simulink model "USV_SASTnewlaw_env"  (R2023a)
settings: Solver=ode4  StartTime=0.0  StopTime=60  FixedStep=0.01  RelTol=1e-3
undefined symbols (not defined in the file or in its folder): sigbuilder_block
libraries: sharedutil x6, simulink_extras x1, aerolibutil x1
(part 1 of 2)
settings Model: Creator=Alex Glz  LastModifiedBy=maxpr
settings SolverCC: ZeroCrossAlgorithm=Adaptive  AlgebraicLoopSolver=TrustRegion
settings DataIOCC: ReturnWorkspaceOutputs=off
settings DebuggingCC: IgnoredZcDiagnostic=none  UnconnectedInputMsg=warning  UnconnectedOutputMsg=warning  UnconnectedLineMsg=warning  PregeneratedLibrarySubsystemCodeDiagnostic=none  ArithmeticOperatorsInVariantConditions=warning
settings ModelReferenceCC: EnableRefExpFcnMdlSchedulingChecks=on
settings SFSimCC: SimUseLocalCustomCode=off  CustomCodeUndefinedFunction=UseInterfaceOnly
settings RTWCC: RTWUseLocalCustomCode=off

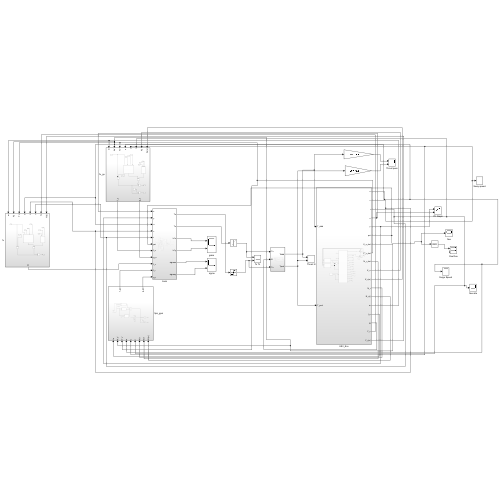
[thumbnail: Simulink's stored preview of the top-level diagram]
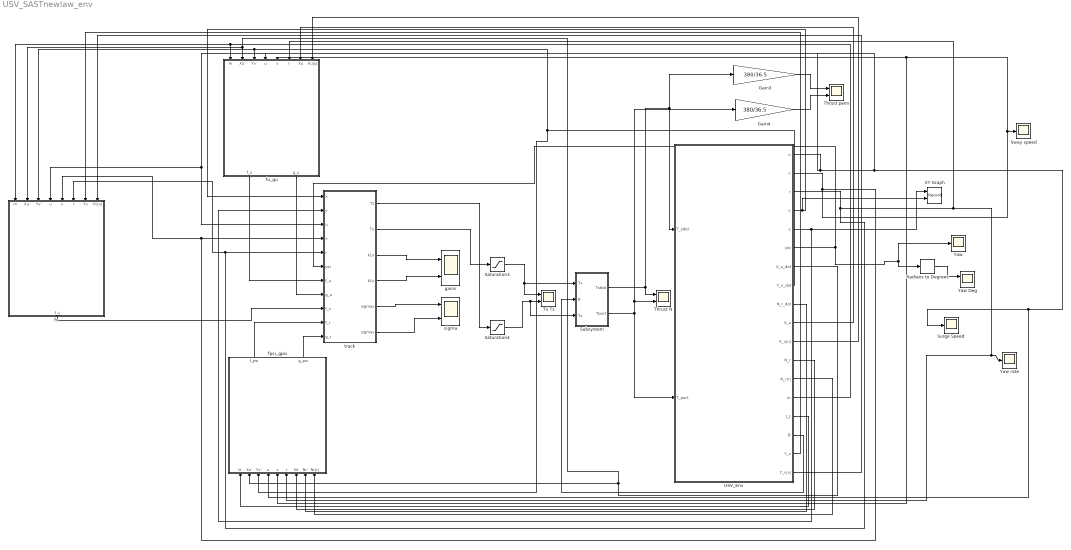
== system USV_SASTnewlaw_env ==
  Gain3 : Gain  Gain=380/36.5
  Gain4 : Gain  Gain=380/36.5
  Radians to Degrees : simulink_extras/Transformations/Radians to Degrees
  Saturation3 : Saturate  UpperLimit=64.97  LowerLimit=-64.97
  Saturation4 : Saturate  UpperLimit=13.31  LowerLimit=-13.31
  Subsystem : Subsystem
  Surge Speed : Scope
  Sway speed : Scope
  Thrust N : Scope  NumInputPorts=2
  Thrust pwm : Scope  NumInputPorts=2
  Tx Tz : Scope  NumInputPorts=2
  USV_Env : Subsystem
  XY Graph : Record  FileSettingsInternal="{\"entries\":[{\"content\":{\"excelSettings\":{\"content\":{},\"type\":\"Streamout.ExcelSettings\"}},\"type\":\"Streamout.FileSettingStorage\",\"uuid\":\"\"}],\"packageUris\":[\"http:\\/\\/schema.mathworks.com\\/mf0\\/streamout_blocks\\/R2020a\"],\"version\":\"1.0\"}"  Layout=[1 1]  SignalsInternal="{\"entries\":[{\"content\":{\"signals\":[{\"content\":{\"blockPath\":[],\"dimensions\":[1],\"domain\":\"\",\"lineColor\":\"#a2142f\",\"plots\":[1],\"port\":1,\"sid\":[\"\"],\"signalID\":306,\"signalName\":\"USV_Env:5\"},\"type\":\"RecordBlkView.Signal\",\"uuid\":\"\"},{\"content\":{\"blockPath\":[],\"dimensions\":[1],\"domain\":\"\",\"lineColor\":\"#139fff\",\"plots\":[1],\"port\":2,\"sid\":[\"\"],\"signalID\":310,\"signalName\":\"USV_Env:4\"},\"type\":\"RecordBlkView.Signal\",\"uuid\":\"\"}]},\"type\":\"RecordBlkView.InputSignals\",\"uuid\":\"\"}],\"packageUris\":[\"http:\\/\\/schema.mathworks.com\\/mf0\\/streamout_blocks\\/R2020a\"],\"version\":\"1.0\"}"  VisualizationBindings="{\"xyplotplugin\":{\"info\":[{\"series\":[{\"bindingParametersList\":[{\"parameter\":\"X-Axis\",\"signalID\":306,\"signalName\":\"USV_Env:5\"},{\"parameter\":\"Y-Axis\",\"signalID\":310,\"signalName\":\"USV_Env:4\"}],\"seriesID\":45570}],\"subplotID\":1}]}}"  CompatibilityTag=XY  st=-1
  Yaw : Scope
  Yaw Deg : Scope  NumInputPorts=2
  Yaw rate : Scope
  fpsi_gpsi : Subsystem
  fu_gu : Subsystem
  fv : Subsystem
  gains : Scope  NumInputPorts=2
  sigma : Scope  NumInputPorts=2
  track : Subsystem
  wires:
  Gain4/1 -> Thrust pwm/2
  Gain3/1 -> Thrust pwm/1
  USV_Env/16(B) -> Subsystem/2(B)
  USV_Env/14(m) -> fv/1(m), fu_gu/1(m)
  USV_Env/7(X_u_dot) -> fv/2(Xu'), fu_gu/2(Xu'), fpsi_gpsi/2(Xu')
  USV_Env/8(Y_v_dot) -> fpsi_gpsi/3(Yv'), fv/3(Yv'), fu_gu/3(Yv')
  USV_Env/1(u) -> fpsi_gpsi/4(u), Surge Speed/1, fu_gu/4(u), track/3(u), fv/4(u)
  USV_Env/2(v) -> fpsi_gpsi/5(v), fu_gu/5(v), Sway speed/1, fv/5(v), track/4(v)
  USV_Env/3(r) -> fv/6(r), track/5(r), fpsi_gpsi/6(r), Yaw rate/1, fu_gu/6(r)
  USV_Env/10(X_u) -> fu_gu/7(Xu)
  USV_Env/11(X_u|u|) -> fu_gu/8(Xu|u|)
  USV_Env/15(I_z) -> fpsi_gpsi/1(Iz)
  USV_Env/12(N_r) -> fpsi_gpsi/7(Nr)
  USV_Env/9(N_r_dot) -> fpsi_gpsi/8(Nr')
  USV_Env/5(y) -> track/2(y), XY Graph/1
  USV_Env/4(x) -> track/1(x), XY Graph/2
  Radians to Degrees/1 -> Yaw Deg/1
  USV_Env/6(psi) -> Yaw/1, Radians to Degrees/1, track/6(psi)
  Saturation4/1 -> Subsystem/3(Tz), Tx Tz/2
  Saturation3/1 -> Subsystem/1(Tx), Tx Tz/1
  Subsystem/2(Tport) -> USV_Env/2(T_port), Thrust N/2, Gain4/1
  Subsystem/1(Tstbd) -> Thrust N/1, USV_Env/1(T_stbd), Gain3/1
  USV_Env/13(N_r|r|) -> fpsi_gpsi/9(Nr|r|)
  track/3(k1x) -> gains/1
  track/4(k1y) -> gains/2
  track/5(sigmax) -> sigma/1
  track/6(sigmay) -> sigma/2
  track/2(Tx) -> Saturation3/1
  track/1(Tz) -> Saturation4/1
  fpsi_gpsi/1(f_psi) -> track/10(f_r)
  fpsi_gpsi/2(g_psi) -> track/11(g_r)
  fu_gu/1(f_u) -> track/7(f_u)
  fu_gu/2(g_u) -> track/8(g_u)
  USV_Env/17(Y_v) -> fv/7(Yv)
  USV_Env/18(Y_v|v|) -> fv/8(Yv|v|)
  fv/1(f_v) -> track/9(f_v)

== system USV_SASTnewlaw_env/Subsystem ==
  Tx : Inport
  B : Inport  Port=2
  Tz : Inport  Port=3
  Gain : Gain  Gain=1/2
  Gain1 : Gain  Gain=1/2
  Product : Product  Inputs=*/
  Product1 : Product  Inputs=*/
  Saturation1 : Saturate  UpperLimit=36.5  LowerLimit=-30
  Saturation2 : Saturate  UpperLimit=36.5  LowerLimit=-30
  Sum : Sum
  Sum1 : Sum  Inputs=+-
  Tstbd : Outport  VectorParamsAs1DForOutWhenUnconnected=off
  Tport : Outport  Port=2  VectorParamsAs1DForOutWhenUnconnected=off
  wires:
  Sum1/1 -> Saturation2/1
  Gain/1 -> Sum/1
  Sum/1 -> Saturation1/1
  B/1 -> Product/2, Product1/2
  Tz/1 -> Product1/1, Product/1
  Saturation1/1 -> Tport/1
  Product/1 -> Sum/2
  Tx/1 -> Gain1/1, Gain/1
  Product1/1 -> Sum1/2
  Saturation2/1 -> Tstbd/1
  Gain1/1 -> Sum1/1

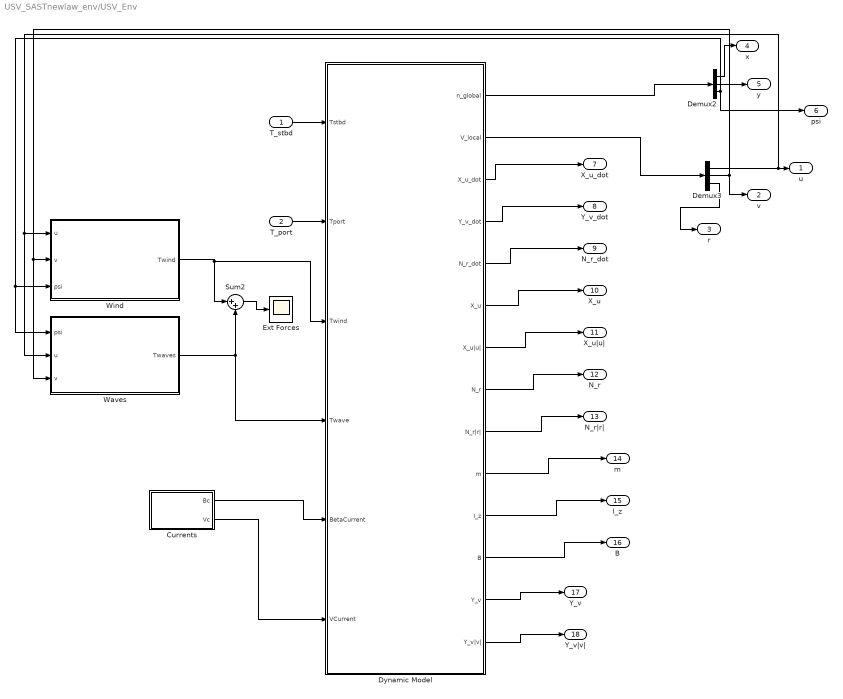
== system USV_SASTnewlaw_env/USV_Env ==
  T_stbd : Inport
  T_port : Inport  Port=2
  Currents : Subsystem
  Demux2 : Demux  Outputs=3
  Demux3 : Demux  Outputs=3
  Dynamic Model : Subsystem
  Ext Forces : Scope
  Sum2 : Sum  Inputs=|++
  Waves : Subsystem
  Wind : Subsystem
  u : Outport
  v : Outport  Port=2
  r : Outport  Port=3
  x : Outport  Port=4
  y : Outport  Port=5
  psi : Outport  Port=6
  X_u_dot : Outport  Port=7  VectorParamsAs1DForOutWhenUnconnected=off
  Y_v_dot : Outport  Port=8  VectorParamsAs1DForOutWhenUnconnected=off
  N_r_dot : Outport  Port=9  VectorParamsAs1DForOutWhenUnconnected=off
  X_u : Outport  Port=10  VectorParamsAs1DForOutWhenUnconnected=off
  X_u|u| : Outport  Port=11  VectorParamsAs1DForOutWhenUnconnected=off
  N_r : Outport  Port=12  VectorParamsAs1DForOutWhenUnconnected=off
  N_r|r| : Outport  Port=13  VectorParamsAs1DForOutWhenUnconnected=off
  m : Outport  Port=14  VectorParamsAs1DForOutWhenUnconnected=off
  I_z : Outport  Port=15  VectorParamsAs1DForOutWhenUnconnected=off
  B : Outport  Port=16  VectorParamsAs1DForOutWhenUnconnected=off
  Y_v : Outport  Port=17  VectorParamsAs1DForOutWhenUnconnected=off
  Y_v|v| : Outport  Port=18  VectorParamsAs1DForOutWhenUnconnected=off
  wires:
  T_stbd/1 -> Dynamic Model/1(Tstbd)
  Currents/1(Bc) -> Dynamic Model/5(BetaCurrent)
  T_port/1 -> Dynamic Model/2(Tport)
  Dynamic Model/2(V_local) -> Demux3/1
  Demux3/2 -> v/1, Waves/3(v), Wind/2(v)
  Demux2/3 -> psi/1, Waves/1(psi), Wind/3(psi)
  Dynamic Model/1(n_global) -> Demux2/1
  Demux3/1 -> u/1, Waves/2(u), Wind/1(u)
  Currents/2(Vc) -> Dynamic Model/6(VCurrent)
  Demux3/3 -> r/1
  Demux2/1 -> x/1
  Demux2/2 -> y/1
  Dynamic Model/3(X_u_dot) -> X_u_dot/1
  Dynamic Model/4(Y_v_dot) -> Y_v_dot/1
  Dynamic Model/5(N_r_dot) -> N_r_dot/1
  Dynamic Model/6(X_u) -> X_u/1
  Dynamic Model/7(X_u|u|) -> X_u|u|/1
  Dynamic Model/8(N_r) -> N_r/1
  Dynamic Model/9(N_r|r|) -> N_r|r|/1
  Dynamic Model/11(I_z) -> I_z/1
  Dynamic Model/10(m) -> m/1
  Dynamic Model/12(B) -> B/1
  Waves/1(Twaves) -> Dynamic Model/4(Twave), Sum2/2
  Wind/1(Twind) -> Dynamic Model/3(Twind), Sum2/1
  Sum2/1 -> Ext Forces/1
  Dynamic Model/13(Y_v) -> Y_v/1
  Dynamic Model/14(Y_v|v|) -> Y_v|v|/1

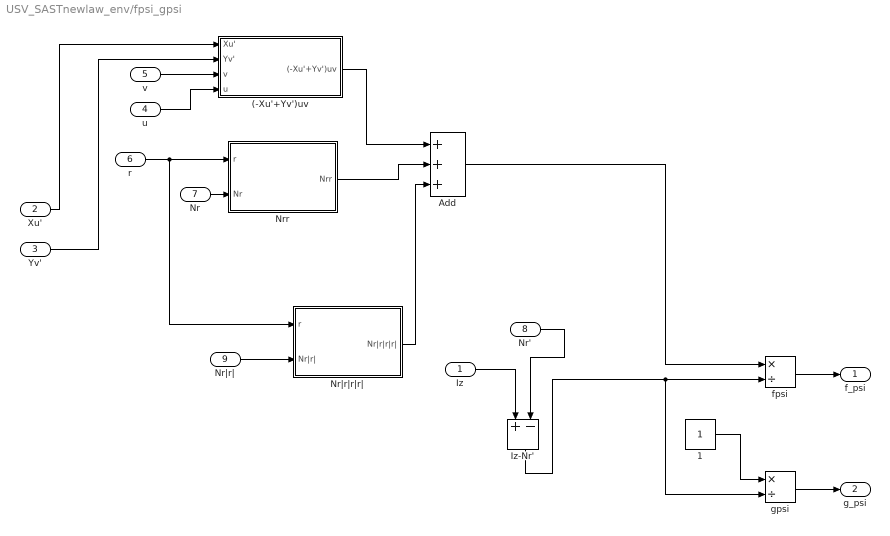
== system USV_SASTnewlaw_env/fpsi_gpsi ==
  Iz : Inport
  Xu' : Inport  Port=2
  Yv' : Inport  Port=3
  u : Inport  Port=4
  v : Inport  Port=5
  r : Inport  Port=6
  Nr : Inport  Port=7
  Nr' : Inport  Port=8
  Nr|r| : Inport  Port=9
  (-Xu'+Yv')uv : Subsystem
  1 : Constant  SampleTime=Inf
  Add : Sum  Inputs=+++
  Iz-Nr' : Sum  Inputs=+-
  Nrr : Subsystem
  Nr|r|r|r| : Subsystem
  fpsi : Product  Inputs=*/
  gpsi : Product  Inputs=*/
  f_psi : Outport  VectorParamsAs1DForOutWhenUnconnected=off
  g_psi : Outport  Port=2  VectorParamsAs1DForOutWhenUnconnected=off
  wires:
  Nr/1 -> Nrr/2(Nr)
  Yv'/1 -> (-Xu'+Yv')uv/2(Yv')
  r/1 -> Nrr/1(r), Nr|r|r|r|/1(r)
  (-Xu'+Yv')uv/1((-Xu'+Yv')uv) -> Add/1
  v/1 -> (-Xu'+Yv')uv/3(v)
  Iz/1 -> Iz-Nr'/1
  Nrr/1(Nrr) -> Add/2
  u/1 -> (-Xu'+Yv')uv/4(u)
  Xu'/1 -> (-Xu'+Yv')uv/1(Xu')
  Nr'/1 -> Iz-Nr'/2
  Nr|r|/1 -> Nr|r|r|r|/2(Nr|r|)
  Nr|r|r|r|/1(Nr|r|r|r|) -> Add/3
  1/1 -> gpsi/1
  gpsi/1 -> g_psi/1
  fpsi/1 -> f_psi/1
  Iz-Nr'/1 -> gpsi/2, fpsi/2
  Add/1 -> fpsi/1

== system USV_SASTnewlaw_env/fu_gu ==
  m : Inport
  Xu' : Inport  Port=2
  Yv' : Inport  Port=3
  u : Inport  Port=4
  v : Inport  Port=5
  r : Inport  Port=6
  Xu : Inport  Port=7
  Xu|u| : Inport  Port=8
  (m-Yv')vr : Subsystem
  1 : Constant  SampleTime=Inf
  Xdrag : Subsystem
  fu : Product  Inputs=*/
  fu*gu : Sum
  gu : Product  Inputs=*/
  m-Xu' : Sum  Inputs=+-
  f_u : Outport  VectorParamsAs1DForOutWhenUnconnected=off
  g_u : Outport  Port=2  VectorParamsAs1DForOutWhenUnconnected=off
  wires:
  Xu/1 -> Xdrag/2(Xu)
  Yv'/1 -> (m-Yv')vr/2(Yv')
  r/1 -> (m-Yv')vr/4(r)
  Xu|u|/1 -> Xdrag/3(Xu|u|)
  m-Xu'/1 -> gu/2, fu/2
  v/1 -> (m-Yv')vr/3(v)
  m/1 -> (m-Yv')vr/1(m), m-Xu'/1
  u/1 -> Xdrag/1(u)
  Xu'/1 -> m-Xu'/2
  (m-Yv')vr/1((m-Yv')vr) -> fu*gu/1
  Xdrag/1(Xdrag) -> fu*gu/2
  fu*gu/1 -> fu/1
  fu/1 -> f_u/1
  gu/1 -> g_u/1
  1/1 -> gu/1

== system USV_SASTnewlaw_env/fv ==
  m : Inport
  Xu' : Inport  Port=2
  Yv' : Inport  Port=3
  u : Inport  Port=4
  v : Inport  Port=5
  r : Inport  Port=6
  Yv : Inport  Port=7
  Yv|v| : Inport  Port=8
  (m-Yv')vr : Subsystem
  Xur + Yuv : Sum
  Ydrag : Subsystem
  fv : Product  Inputs=*/
  m-Yv' : Sum  Inputs=+-
  f_v : Outport  VectorParamsAs1DForOutWhenUnconnected=off
  wires:
  Yv/1 -> Ydrag/2(Yv)
  Yv'/1 -> m-Yv'/2
  r/1 -> (m-Yv')vr/4(r)
  Yv|v|/1 -> Ydrag/3(Yv|v|)
  m-Yv'/1 -> fv/2
  v/1 -> Ydrag/1(v)
  m/1 -> (m-Yv')vr/1(m), m-Yv'/1
  u/1 -> (m-Yv')vr/3(u)
  Xu'/1 -> (m-Yv')vr/2(Xu')
  fv/1 -> f_v/1
  Xur + Yuv/1 -> fv/1
  (m-Yv')vr/1((-m+Xu')ur) -> Xur + Yuv/1
  Ydrag/1(Ydrag) -> Xur + Yuv/2

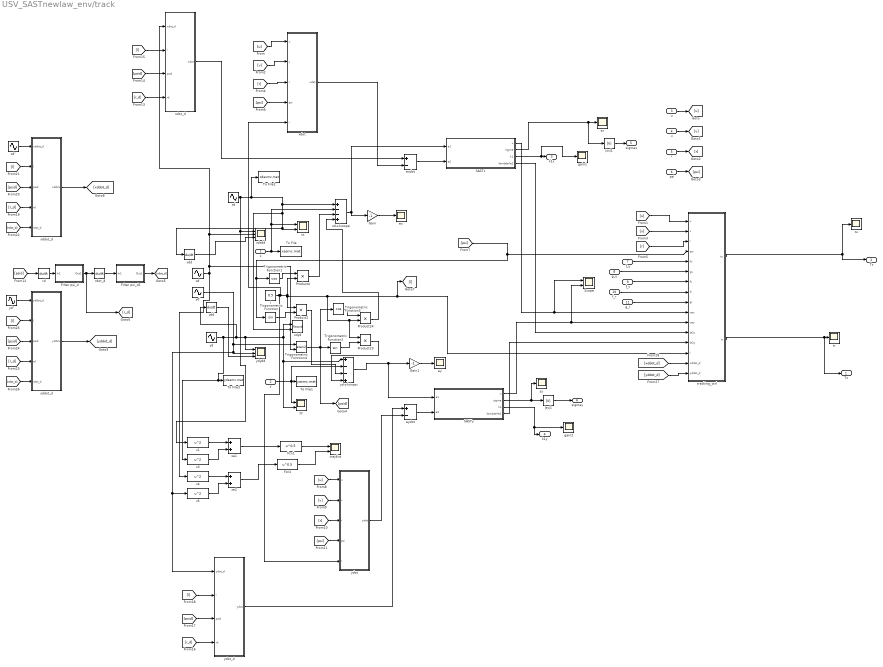
== system USV_SASTnewlaw_env/track ==
  x : Inport
  y : Inport  Port=2
  u : Inport  Port=3
  v : Inport  Port=4
  r : Inport  Port=5
  psi : Inport  Port=6
  f_u : Inport  Port=7
  g_u : Inport  Port=8
  f_v : Inport  Port=9
  f_r : Inport  Port=10
  g_r : Inport  Port=11
  Fcn1 : Fcn  Expr=u^0.5
  Fcn2 : Fcn  Expr=u^0.5
  Filter psi_d : Subsystem
  Filter psi_d1 : Subsystem
  Gain : Gain  Gain=-1
  Gain1 : Gain  Gain=-1
  Product{2,4,23..24} (4 alike) : Product
  SASTx : Subsystem
  SASTy : Subsystem
  Scope : Scope  NumInputPorts=2
  To File : ToFile  Filename=xasmc.mat
  To File1 : ToFile  Filename=yasmc.mat
  To File2 : ToFile  Filename=xdasmc.mat
  To File3 : ToFile  Filename=ydasmc.mat
  Trigonometric Function : Trigonometry
  Trigonometric Function1 : Trigonometry  Operator=cos
  Trigonometric Function2 : Trigonometry
  Trigonometric Function3 : Trigonometry  Operator=cos
  Trigonometric Function4 : Trigonometry  Operator=atan2
  ex : Scope
  exdot : Sum  Inputs=+-
  ey : Scope
  eydot : Sum  Inputs=+-
  gain1 : Scope
  gain2 : Scope
  l : Constant  Value=0.5
  rd : Derivative
  rdot_d : Derivative
  sx : Scope
  sy : Scope
  tr : Scope
  tracking_ctrl : MATLAB Function  TreatAsAtomicUnit=on
  trajdist : Scope  NumInputPorts=2
  tu : Scope
  v{1,3..5} (4 alike) : Fcn  Expr=u^2
  xd : Sin  Amplitude=2.5  Bias=0.5  Frequency=pi/15  SampleTime=0
  xd' : Sin  Amplitude=2.5*pi/15  Frequency=pi/15  Phase=pi/2  SampleTime=0
  xd'' : Sin  Amplitude=-2.5*(pi/15)*(pi/15)  Frequency=pi/15  SampleTime=0
  xd-x-lcospsi : Sum  Inputs=+--+
  xdd : Derivative
  xddot_d : MATLAB Function  TreatAsAtomicUnit=on
  xdot : MATLAB Function  TreatAsAtomicUnit=on
  xdot_d : MATLAB Function  TreatAsAtomicUnit=on
  xdxdd : Scope  NumInputPorts=3
  xdyd : Record  FileSettingsInternal="{\"entries\":[{\"content\":{\"excelSettings\":{\"content\":{},\"type\":\"Streamout.ExcelSettings\"}},\"type\":\"Streamout.FileSettingStorage\",\"uuid\":\"\"}],\"packageUris\":[\"http:\\/\\/schema.mathworks.com\\/mf0\\/streamout_blocks\\/R2020a\"],\"version\":\"1.0\"}"  Layout=[1 1]  SignalsInternal="{\"entries\":[{\"content\":{\"signals\":[{\"content\":{\"blockPath\":[],\"dimensions\":[1],\"domain\":\"\",\"lineColor\":\"#a2142f\",\"plots\":[1],\"port\":1,\"sid\":[\"\"],\"signalID\":395,\"signalName\":\"yd\"},\"type\":\"RecordBlkView.Signal\",\"uuid\":\"\"},{\"content\":{\"blockPath\":[],\"dimensions\":[1],\"domain\":\"\",\"lineColor\":\"#139fff\",\"plots\":[1],\"port\":2,\"sid\":[\"\"],\"signalID\":399,\"signalName\":\"xd\"},\"type\":\"RecordBlkView.Signal\",\"uuid\":\"\"}]},\"type\":\"RecordBlkView.InputSignals\",\"uuid\":\"\"}],\"packageUris\":[\"http:\\/\\/schema.mathworks.com\\/mf0\\/streamout_blocks\\/R2020a\"],\"version\":\"1.0\"}"  VisualizationBindings="{\"xyplotplugin\":{\"info\":[{\"series\":[{\"bindingParametersList\":[{\"parameter\":\"X-Axis\",\"signalID\":395,\"signalName\":\"yd\"},{\"parameter\":\"Y-Axis\",\"signalID\":399,\"signalName\":\"xd\"}],\"seriesID\":16886}],\"subplotID\":1}]}}"  CompatibilityTag=XY  st=-1
  xe1 : Sum
  xe2 : Sum
  xx : Scope  NumInputPorts=2
  yd : Sin  Amplitude=7  Bias=-7.5  Frequency=pi/30  Phase=pi/2  SampleTime=0
  yd' : Sin  Amplitude=-7*pi/30  Frequency=pi/30  SampleTime=0
  yd'' : Sin  Amplitude=-7*(pi/30)*(pi/30)  Frequency=pi/30  Phase=pi/2  SampleTime=0
  yd-y-lsinpsi : Sum  Inputs=+--+
  ydd : Derivative
  yddot_d : MATLAB Function  TreatAsAtomicUnit=on
  ydot : MATLAB Function  TreatAsAtomicUnit=on
  ydot_d : MATLAB Function  TreatAsAtomicUnit=on
  ydydd : Scope  NumInputPorts=3
  yy : Scope  NumInputPorts=2
  |sx|1 : Abs  SaturateOnIntegerOverflow=off
  |sy|1 : Abs  SaturateOnIntegerOverflow=off
  Tz : Outport
  Tx : Outport  Port=2
  k1x : Outport  Port=3  VectorParamsAs1DForOutWhenUnconnected=off
  k1y : Outport  Port=4  VectorParamsAs1DForOutWhenUnconnected=off
  sigmax : Outport  Port=5  VectorParamsAs1DForOutWhenUnconnected=off
  sigmay : Outport  Port=6  VectorParamsAs1DForOutWhenUnconnected=off
  wires:
  tracking_ctrl/2(tr) -> Tz/1, tr/1
  y/1 -> yd-y-lsinpsi/2, To File1/1, yy/1
  x/1 -> xd-x-lcospsi/2, xx/1, To File/1
  xd/1 -> v1/1, xdxdd/1, To File2/1, xd-x-lcospsi/1, xx/2, xdd/1, xdyd/2
  yd/1 -> v3/1, To File3/1, yd-y-lsinpsi/1, yy/2, xdyd/1, ydydd/1, ydd/1
  xd-x-lcospsi/1 -> SASTx/1(e1), Gain/1
  yd'/1 -> ydydd/2, ydot_d/1(ydot_d), v5/1, Trigonometric Function4/1
  xd'/1 -> xdot_d/1(xdot_d), xdxdd/2, Trigonometric Function4/2, v4/1
  tracking_ctrl/1(tu) -> tu/1, Tx/1
  ydd/1 -> ydydd/3
  xdd/1 -> xdxdd/3
  Fcn1/1 -> trajdist/1
  Fcn2/1 -> trajdist/2
  xe1/1 -> Fcn1/1
  v1/1 -> xe1/1
  v3/1 -> xe1/2
  xe2/1 -> Fcn2/1
  v4/1 -> xe2/1
  v5/1 -> xe2/2
  yd-y-lsinpsi/1 -> SASTy/1(e1), Gain1/1
  Product2/1 -> yd-y-lsinpsi/3
  Product4/1 -> xd-x-lcospsi/3
  [psi] -> tracking_ctrl/4(psi), Trigonometric Function1/1, Trigonometric Function/1
  Trigonometric Function1/1 -> Product4/1
  Trigonometric Function/1 -> Product2/2
  SASTx/2(sigma) -> |sx|1/1, sx/1
  |sy|1/1 -> sigmay/1
  |sx|1/1 -> sigmax/1
  Trigonometric Function4/1 -> Trigonometric Function3/1, Trigonometric Function2/1, [psid]
  Trigonometric Function2/1 -> Product23/2
  Trigonometric Function3/1 -> Product24/1
  Product23/1 -> yd-y-lsinpsi/4
  Product24/1 -> xd-x-lcospsi/4
  SASTx/3(k1) -> gain1/1, k1x/1
  SASTy/2(sigma) -> sy/1, |sy|1/1
  SASTy/3(k1) -> k1y/1, gain2/1
  u/1 -> [u]
  [v] -> tracking_ctrl/2(v)
  [r] -> tracking_ctrl/3(r)
  f_u/1 -> tracking_ctrl/5(fu)
  g_u/1 -> tracking_ctrl/6(gu)
  f_v/1 -> tracking_ctrl/7(fv)
  f_r/1 -> tracking_ctrl/8(fr)
  g_r/1 -> tracking_ctrl/9(gr)
  SASTx/1(u) -> tracking_ctrl/10(uax), Scope/1
  SASTy/1(u) -> tracking_ctrl/11(uay), Scope/2
  SASTx/4(lambda*e2) -> tracking_ctrl/12(le2x)
  SASTy/4(lambda*e2) -> tracking_ctrl/13(le2y)
  eydot/1 -> SASTy/2(e2)
  exdot/1 -> SASTx/2(e2)
  xdot/1(xdot) -> exdot/2
  [u] -> xdot/1(u)
  [u] -> tracking_ctrl/1(u)
  psi/1 -> [psi]
  v/1 -> [v]
  r/1 -> [r]
  [v] -> xdot/2(v)
  [r] -> xdot/3(r)
  [psi] -> xdot/4(psi)
  ydot/1(ydot) -> eydot/2
  [r] -> ydot/3(r)
  l/1 -> ydot/5(l), xdot/5(l), [l], tracking_ctrl/14(l), Product23/1, Product24/2, Product2/1, Product4/2
  [v] -> ydot/2(v)
  [psi] -> ydot/4(psi)
  [u] -> ydot/1(u)
  xdot_d/1(xdot) -> exdot/1
  [psid] -> rd/1
  rd/1 -> Filter psi_d/1(In1)
  rdot_d/1 -> Filter psi_d1/1(In1)
  [r_d] -> xdot_d/4(rd)
  [psid] -> xdot_d/3(psid)
  [l] -> xdot_d/2(l)
  ydot_d/1(ydot) -> eydot/1
  [l] -> ydot_d/2(l)
  [r_d] -> ydot_d/4(rd)
  [psid] -> ydot_d/3(psid)
  xd''/1 -> xddot_d/1(xddot_d)
  [l] -> xddot_d/2(l)
  [psid] -> xddot_d/3(psid)
  [r_d] -> xddot_d/4(rd)
  [rdot_d] -> xddot_d/5(rdot_d)
  xddot_d/1(xddot) -> [xddot_d]
  yddot_d/1(yddot) -> [yddot_d]
  [psid] -> yddot_d/3(psid)
  [l] -> yddot_d/2(l)
  [r_d] -> yddot_d/4(rd)
  [rdot_d] -> yddot_d/5(rdot_d)
  yd''/1 -> yddot_d/1(yddot_d)
  [yddot_d] -> tracking_ctrl/16(yddot_d)
  [xddot_d] -> tracking_ctrl/15(xddot_d)
  Filter psi_d/1(Out1) -> rdot_d/1, [r_d]
  Filter psi_d1/1(Out1) -> [rdot_d]
  Gain/1 -> ex/1
  Gain1/1 -> ey/1

== system USV_SASTnewlaw_env/USV_Env/Currents ==
  Beta : Constant  Value=0.8
  Current Speed : Scope
  Product : Product
  Saturation : Saturate  UpperLimit=1  LowerLimit=-1
  Sum : Sum  Inputs=+-
  Vc_int : Integrator
  gamawr : Gain  Gain=.5
  mu : Constant  Value=0.5
  w : Subsystem  Tag=STV Subsys  LoadFcn=sigbuilder_block('load');  StartFcn=sigbuilder_block('start');  StopFcn=sigbuilder_block('stop');  ClipboardFcn=sigbuilder_block('clipboard');  mask(Sigbuilder block){tuvar=[0:10]}
      mask help: Simulink:masks:SigbuilderBlock_MD
      mask init:
      | if ~strcmp(get_param(bdroot(gcbh),'SimulationStatus'),'stopped') tuvar = sigbuilder_block('maskInit'); end
      settings: CopyFcn=sigbuilder_block('copy');  DeleteFcn=sigbuilder_block('delete');  ModelCloseFcn=sigbuilder_block('modelClose');  PreSaveFcn=sigbuilder_block('preSave');  PauseFcn=sigbuilder_block('pause');  ContinueFcn=sigbuilder_block('continue');  NameChangeFcn=sigbuilder_block('namechange');  OpenFcn=sigbuilder_block('open',[86.25 30 718.5 658.5 ]);  CloseFcn=sigbuilder_block('close');
      mask Display: plot(0, 0, 100, 100,[2, 2, 32, 32, 2], [68, 8, 8, 68, 68],[32, 2], [38, 38], [32, 19, 2],[53, 60, 44], [32, 17, 17, 2],[16, 16, 31, 31]);txt = getActiveGroup(gcbh);text(2, 100, txt,'verticalAlignment', 'top');
  Bc : Outport  VectorParamsAs1DForOutWhenUnconnected=off
  Vc : Outport  Port=2  VectorParamsAs1DForOutWhenUnconnected=off
  wires:
  w/1(white_noise) -> Sum/1
  Product/1 -> Sum/2
  Sum/1 -> Vc_int/1
  mu/1 -> Product/1
  Beta/1 -> Bc/1
  Vc_int/1 -> Saturation/1, Product/2
  Saturation/1 -> gamawr/1, Current Speed/1
  gamawr/1 -> Vc/1

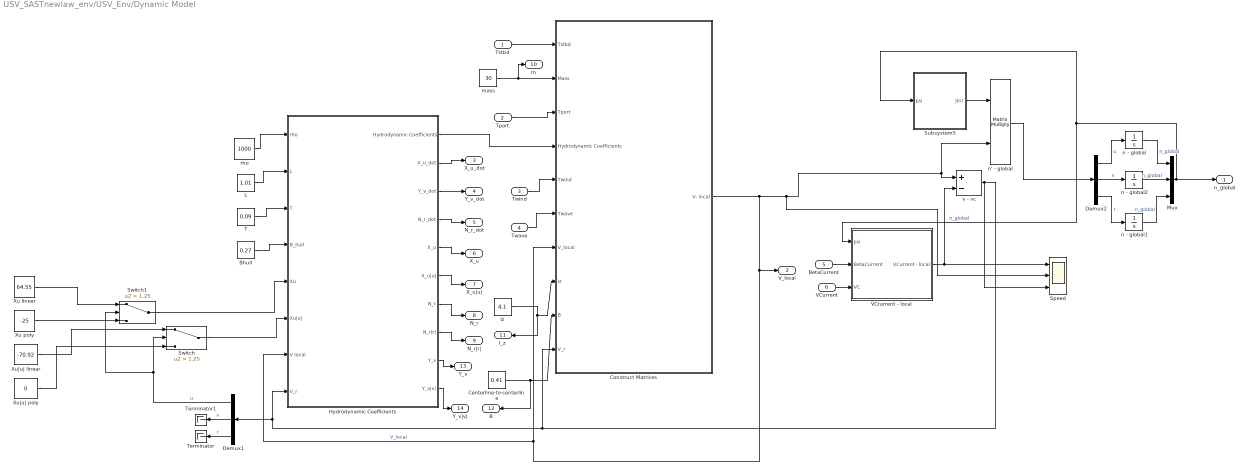
== system USV_SASTnewlaw_env/USV_Env/Dynamic Model ==
  Tstbd : Inport
  Tport : Inport  Port=2
  Twind : Inport  Port=3
  Twave : Inport  Port=4
  BetaCurrent : Inport  Port=5
  VCurrent : Inport  Port=6
  "Bhull " : Constant  Value=0.27
  Centerline-to-centerline : Constant  Value=0.41
  Construct Matrices : Subsystem
  Demux1 : Demux  Outputs=3
  Demux2 : Demux  Outputs=3
  Hydrodynamic Coefficients : Subsystem
  Iz : Constant  Value=4.1
  L : Constant  Value=1.01
  Mux : Mux  Inputs=3
  Speed : Scope  NumInputPorts=3
  Subsystem5 : Subsystem
  Switch : Switch  Criteria=u2 > Threshold  Threshold=1.25  SaturateOnIntegerOverflow=off  InputSameDT=off
  Switch1 : Switch  Criteria=u2 > Threshold  Threshold=1.25  SaturateOnIntegerOverflow=off  InputSameDT=off
  T : Constant  Value=0.09
  Terminator : Terminator
  Terminator1 : Terminator
  VCrurrent - local : Subsystem
  Xu linear : Constant  Value=64.55
  Xu poly : Constant  Value=-25
  Xu|u| linear : Constant  Value=-70.92
  Xu|u| poly : Constant  Value=0
  mass : Constant  Value=30
  n - global : Integrator
  n - global1 : Integrator  WrapState=on
  n - global2 : Integrator
  n' - global : Product  Multiplication=Matrix(*)
  rho : Constant  Value=1000
  v - vc : Sum  Inputs=+-
  n_global : Outport  VectorParamsAs1DForOutWhenUnconnected=off
  V_local : Outport  Port=2  VectorParamsAs1DForOutWhenUnconnected=off
  X_u_dot : Outport  Port=3  VectorParamsAs1DForOutWhenUnconnected=off
  Y_v_dot : Outport  Port=4  VectorParamsAs1DForOutWhenUnconnected=off
  N_r_dot : Outport  Port=5  VectorParamsAs1DForOutWhenUnconnected=off
  X_u : Outport  Port=6  VectorParamsAs1DForOutWhenUnconnected=off
  X_u|u| : Outport  Port=7  VectorParamsAs1DForOutWhenUnconnected=off
  N_r : Outport  Port=8  VectorParamsAs1DForOutWhenUnconnected=off
  N_r|r| : Outport  Port=9  VectorParamsAs1DForOutWhenUnconnected=off
  m : Outport  Port=10  VectorParamsAs1DForOutWhenUnconnected=off
  I_z : Outport  Port=11  VectorParamsAs1DForOutWhenUnconnected=off
  B : Outport  Port=12  VectorParamsAs1DForOutWhenUnconnected=off
  Y_v : Outport  Port=13  VectorParamsAs1DForOutWhenUnconnected=off
  Y_v|v| : Outport  Port=14  VectorParamsAs1DForOutWhenUnconnected=off
  wires:
  Mux/1 -> Subsystem5/1(psi), VCrurrent - local/1(psi), n_global/1  "n_global"
  Construct Matrices/1(V- local) -> V_local/1, Construct Matrices/7(V_local), Hydrodynamic Coefficients/7(V local), v - vc/1, n' - global/2, Speed/2  "V_local"
  n' - global/1 -> Demux2/1
  Subsystem5/1(J(n)) -> n' - global/1
  rho/1 -> Hydrodynamic Coefficients/1(rho)
  L/1 -> Hydrodynamic Coefficients/2(L)
  Tport/1 -> Construct Matrices/3(Tport)
  Tstbd/1 -> Construct Matrices/1(Tstbd)
  mass/1 -> m/1, Construct Matrices/2("Mass ")
  Hydrodynamic Coefficients/1("Hydrodynamic Coefficients ") -> Construct Matrices/4(Hydrodynamic Coefficients)
  T/1 -> Hydrodynamic Coefficients/3(T)
  "Bhull "/1 -> Hydrodynamic Coefficients/4(B_hull)
  Switch/1 -> Hydrodynamic Coefficients/6(Xu|u|)
  Demux1/1 -> Switch1/2, Switch/2  "u"
  Xu|u| poly/1 -> Switch/3
  Xu|u| linear/1 -> Switch/1
  Switch1/1 -> Hydrodynamic Coefficients/5(Xu)
  Xu poly/1 -> Switch1/3
  Xu linear/1 -> Switch1/1
  Demux1/3 -> Terminator/1  "r"
  Demux1/2 -> Terminator1/1  "v"
  Twave/1 -> Construct Matrices/6(Twave)
  Twind/1 -> Construct Matrices/5(Twind)
  BetaCurrent/1 -> VCrurrent - local/2(BetaCurrent)
  VCrurrent - local/1(VCurrent - local) -> v - vc/2, Speed/1
  v - vc/1 -> Speed/3, Construct Matrices/10(V_r), Hydrodynamic Coefficients/8(V_r), Demux1/1
  VCurrent/1 -> VCrurrent - local/3(VC)
  Hydrodynamic Coefficients/2(X_u_dot) -> X_u_dot/1
  Hydrodynamic Coefficients/3(Y_v_dot) -> Y_v_dot/1
  Hydrodynamic Coefficients/4(N_r_dot) -> N_r_dot/1
  Hydrodynamic Coefficients/5(X_u) -> X_u/1
  Hydrodynamic Coefficients/6(X_u|u|) -> X_u|u|/1
  Hydrodynamic Coefficients/7(N_r) -> N_r/1
  Hydrodynamic Coefficients/8(N_r|r|) -> N_r|r|/1
  Iz/1 -> Construct Matrices/8(Iz), I_z/1
  Centerline-to-centerline/1 -> Construct Matrices/9(B), B/1
  Demux2/3 -> n - global1/1  "r"
  n - global1/1 -> Mux/3  "n_global"
  Demux2/1 -> n - global/1  "u"
  n - global/1 -> Mux/1  "n_global"
  Demux2/2 -> n - global2/1  "v"
  n - global2/1 -> Mux/2  "n_global"
  Hydrodynamic Coefficients/9(Y_v) -> Y_v/1
  Hydrodynamic Coefficients/10(Y_v|v|) -> Y_v|v|/1

== system USV_SASTnewlaw_env/USV_Env/Waves ==
  psi : Inport
  u : Inport  Port=2
  v : Inport  Port=3
  Fwave : Subsystem
  Mux : Mux  Inputs=3
  N : Subsystem
  Product1 : Product
  Product2 : Product
  Sum7 : Sum  Inputs=|+-
  Trigonometric Function : Trigonometry
  Trigonometric Function1 : Trigonometry  Operator=cos
  Wave Force : Scope
  lambda : Constant  Value=0.1
  wave_dir : Constant
  we : Subsystem
  Twaves : Outport  VectorParamsAs1DForOutWhenUnconnected=off
  wires:
  Mux/1 -> Wave Force/1, Twaves/1  "T"
  N/1(Nwave) -> Mux/3
  we/1(w) -> Fwave/1(we), N/1(we)
  v/1 -> we/3(v)
  u/1 -> we/2(u)
  lambda/1 -> N/2(lambda), Fwave/2(lambda)
  Fwave/1(Xwave) -> Product1/1, Product2/2
  Trigonometric Function/1 -> Product1/2
  Trigonometric Function1/1 -> Product2/1
  Product1/1 -> Mux/2
  wave_dir/1 -> we/4(wave_beta), Sum7/1
  Sum7/1 -> Trigonometric Function1/1, Trigonometric Function/1
  Product2/1 -> Mux/1
  psi/1 -> Sum7/2, we/1(psi)

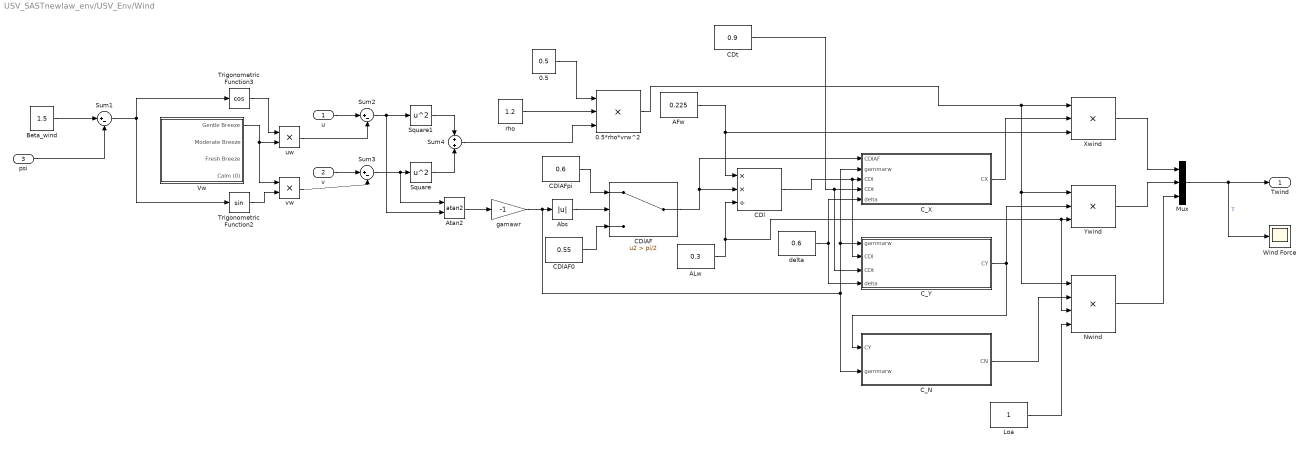
== system USV_SASTnewlaw_env/USV_Env/Wind ==
  u : Inport
  v : Inport  Port=2
  psi : Inport  Port=3
  0.5 : Constant  Value=0.5
  0.5*rho*vrw^2 : Product  Inputs=3
  AFw : Constant  Value=0.225
  ALw : Constant  Value=0.3
  Abs : Abs  ZeroCross=off  SaturateOnIntegerOverflow=off
  Atan2 : Trigonometry  Operator=atan2
  Beta_wind : Constant  Value=1.5
  CDl : Product  Inputs=**/
  CDlAF : Switch  Criteria=u2 > Threshold  Threshold=pi/2  ZeroCross=off  SaturateOnIntegerOverflow=off  InputSameDT=off
  CDlAF0 : Constant  Value=0.55
  CDlAFpi : Constant  Value=0.6
  CDt : Constant  Value=0.9
  C_N : Subsystem
  C_X : Subsystem
  C_Y : Subsystem
  Loa : Constant
  Mux : Mux  Inputs=3
  Nwind : Product  Inputs=4
  Square : Math  Operator=square
  Square1 : Math  Operator=square
  Sum1 : Sum  Inputs=|+-
  Sum2 : Sum  Inputs=|+-
  Sum3 : Sum  Inputs=|+-
  Sum4 : Sum
  Trigonometric Function2 : Trigonometry
  Trigonometric Function3 : Trigonometry  Operator=cos
  Vw : Subsystem  Tag=STV Subsys  LoadFcn=sigbuilder_block('load');  StartFcn=sigbuilder_block('start');  StopFcn=sigbuilder_block('stop');  ClipboardFcn=sigbuilder_block('clipboard');  mask(Sigbuilder block){tuvar=[0:10]}
      mask help: Simulink:masks:SigbuilderBlock_MD
      mask init:
      | if ~strcmp(get_param(bdroot(gcbh),'SimulationStatus'),'stopped') tuvar = sigbuilder_block('maskInit'); end
      settings: CopyFcn=sigbuilder_block('copy');  DeleteFcn=sigbuilder_block('delete');  ModelCloseFcn=sigbuilder_block('modelClose');  PreSaveFcn=sigbuilder_block('preSave');  PauseFcn=sigbuilder_block('pause');  ContinueFcn=sigbuilder_block('continue');  NameChangeFcn=sigbuilder_block('namechange');  OpenFcn=sigbuilder_block('open',[48.75 0 1391.25 628.5 ]);  CloseFcn=sigbuilder_block('close');
      mask Display: plot(0, 0, 100, 100,[2, 2, 32, 32, 2], [68, 8, 8, 68, 68],[32, 2], [38, 38], [32, 19, 2],[53, 60, 44], [32, 17, 17, 2],[16, 16, 31, 31]);txt = getActiveGroup(gcbh);text(2, 100, txt,'verticalAlignment', 'top');
  Wind Force : Scope
  Xwind : Product  Inputs=3
  Ywind : Product  Inputs=3
  delta : Constant  Value=0.6
  gamawr : Gain  Gain=-1
  rho : Constant  Value=1.2
  uw : Product
  vw : Product
  Twind : Outport  VectorParamsAs1DForOutWhenUnconnected=off
  wires:
  Mux/1 -> Wind Force/1, Twind/1  "T"
  u/1 -> Sum2/1
  Trigonometric Function2/1 -> vw/2
  vw/1 -> Sum3/2
  Trigonometric Function3/1 -> uw/1
  uw/1 -> Sum2/2
  Vw/1(Gentle Breeze) -> vw/1, uw/2
  Sum1/1 -> Trigonometric Function3/1, Trigonometric Function2/1
  Beta_wind/1 -> Sum1/1
  v/1 -> Sum3/1
  psi/1 -> Sum1/2
  Square/1 -> Sum4/2
  Sum3/1 -> Atan2/1, Square/1
  Sum4/1 -> 0.5*rho*vrw^2/3
  Square1/1 -> Sum4/1
  Sum2/1 -> Square1/1, Atan2/2
  Atan2/1 -> gamawr/1
  rho/1 -> 0.5*rho*vrw^2/2
  0.5/1 -> 0.5*rho*vrw^2/1
  gamawr/1 -> C_N/2(gammarw), C_Y/1(gammarw), C_X/2(gammarw), Abs/1
  Abs/1 -> CDlAF/2
  CDlAFpi/1 -> CDlAF/1
  CDlAF0/1 -> CDlAF/3
  AFw/1 -> Xwind/3, CDl/1
  ALw/1 -> Nwind/3, Ywind/3, CDl/3
  CDlAF/1 -> CDl/2, C_X/1(CDlAF)
  CDl/1 -> C_Y/2(CDl), C_X/3(CDl)
  CDt/1 -> C_X/4(CDt), C_Y/3(CDt)
  delta/1 -> C_Y/4(delta), C_X/5(delta)
  C_Y/1(CY) -> Ywind/2, C_N/1(CY)
  0.5*rho*vrw^2/1 -> Nwind/1, Ywind/1, Xwind/1
  C_X/1(CX) -> Xwind/2
  C_N/1(CN) -> Nwind/2
  Loa/1 -> Nwind/4
  Xwind/1 -> Mux/1
  Ywind/1 -> Mux/2
  Nwind/1 -> Mux/3

== system USV_SASTnewlaw_env/fpsi_gpsi/(-Xu'+Yv')uv ==
  Xu' : Inport
  Yv' : Inport  Port=2
  v : Inport  Port=3
  u : Inport  Port=4
  -Xu'+Yv' : Sum  Inputs=-+
  Product : Product  Inputs=3
  (-Xu'+Yv')uv : Outport  VectorParamsAs1DForOutWhenUnconnected=off
  wires:
  Yv'/1 -> -Xu'+Yv'/2
  v/1 -> Product/3
  -Xu'+Yv'/1 -> Product/1
  u/1 -> Product/2
  Product/1 -> (-Xu'+Yv')uv/1
  Xu'/1 -> -Xu'+Yv'/1

== system USV_SASTnewlaw_env/fpsi_gpsi/Nrr ==
  r : Inport
  Nr : Inport  Port=2
  Product1 : Product
  Nrr : Outport  VectorParamsAs1DForOutWhenUnconnected=off
  wires:
  Product1/1 -> Nrr/1
  Nr/1 -> Product1/1
  r/1 -> Product1/2

== system USV_SASTnewlaw_env/fpsi_gpsi/Nr|r|r|r| ==
  r : Inport
  Nr|r| : Inport  Port=2
  Abs : Abs  SaturateOnIntegerOverflow=off
  Product1 : Product  Inputs=3
  Nr|r|r|r| : Outport  VectorParamsAs1DForOutWhenUnconnected=off
  wires:
  Product1/1 -> Nr|r|r|r|/1
  Nr|r|/1 -> Product1/1
  r/1 -> Abs/1, Product1/2
  Abs/1 -> Product1/3

== system USV_SASTnewlaw_env/fu_gu/(m-Yv')vr ==
  m : Inport
  Yv' : Inport  Port=2
  v : Inport  Port=3
  r : Inport  Port=4
  Product : Product  Inputs=3
  m-Yv' : Sum  Inputs=+-
  (m-Yv')vr : Outport  VectorParamsAs1DForOutWhenUnconnected=off
  wires:
  Yv'/1 -> m-Yv'/2
  v/1 -> Product/2
  m-Yv'/1 -> Product/1
  r/1 -> Product/3
  Product/1 -> (m-Yv')vr/1
  m/1 -> m-Yv'/1

== system USV_SASTnewlaw_env/fu_gu/Xdrag ==
  u : Inport
  Xu : Inport  Port=2
  Xu|u| : Inport  Port=3
  Abs : Abs  SaturateOnIntegerOverflow=off
  Add : Sum
  Product : Product  Inputs=3
  Product1 : Product
  Xdrag : Outport  VectorParamsAs1DForOutWhenUnconnected=off
  wires:
  Add/1 -> Xdrag/1
  Xu|u|/1 -> Product/1
  Product/1 -> Add/1
  Xu/1 -> Product1/1
  Product1/1 -> Add/2
  Abs/1 -> Product1/2, Product/2
  u/1 -> Product/3, Abs/1

== system USV_SASTnewlaw_env/fv/(m-Yv')vr ==
  m : Inport
  Xu' : Inport  Port=2
  u : Inport  Port=3
  r : Inport  Port=4
  -m+Xu' : Sum  Inputs=-+
  Product : Product  Inputs=3
  (-m+Xu')ur : Outport  VectorParamsAs1DForOutWhenUnconnected=off
  wires:
  Xu'/1 -> -m+Xu'/2
  u/1 -> Product/2
  -m+Xu'/1 -> Product/1
  r/1 -> Product/3
  Product/1 -> (-m+Xu')ur/1
  m/1 -> -m+Xu'/1

== system USV_SASTnewlaw_env/fv/Ydrag ==
  v : Inport
  Yv : Inport  Port=2
  Yv|v| : Inport  Port=3
  Abs : Abs  SaturateOnIntegerOverflow=off
  Add : Sum
  Product : Product  Inputs=3
  Product1 : Product
  Ydrag : Outport  VectorParamsAs1DForOutWhenUnconnected=off
  wires:
  Add/1 -> Ydrag/1
  Yv|v|/1 -> Product/1
  Product/1 -> Add/1
  Yv/1 -> Product1/1
  Product1/1 -> Add/2
  Abs/1 -> Product1/2, Product/2
  v/1 -> Product/3, Abs/1

== system USV_SASTnewlaw_env/track/Filter psi_d ==
  In1 : Inport
  Gain2 : Gain  Gain=7
  Gain5 : Gain  Gain=7
  Gain7 : Gain
  Gain8 : Gain  Gain=2
  Integrator2 : Integrator
  Integrator3 : Integrator
  Sum12 : Sum  Inputs=|+-
  Sum13 : Sum  Inputs=|+-
  Out1 : Outport  VectorParamsAs1DForOutWhenUnconnected=off
  wires:
  Gain7/1 -> Gain8/1
  Sum12/1 -> Gain2/1
  Integrator3/1 -> Out1/1, Sum12/2
  In1/1 -> Sum12/1
  Gain2/1 -> Sum13/1
  Gain5/1 -> Integrator2/1
  Sum13/1 -> Gain5/1
  Gain8/1 -> Sum13/2
  Integrator2/1 -> Gain7/1, Integrator3/1

== system USV_SASTnewlaw_env/track/Filter psi_d1 ==
  In1 : Inport
  Gain2 : Gain  Gain=7
  Gain5 : Gain  Gain=7
  Gain7 : Gain
  Gain8 : Gain  Gain=2
  Integrator2 : Integrator
  Integrator3 : Integrator
  Sum12 : Sum  Inputs=|+-
  Sum13 : Sum  Inputs=|+-
  Out1 : Outport  VectorParamsAs1DForOutWhenUnconnected=off
  wires:
  Gain7/1 -> Gain8/1
  Sum12/1 -> Gain2/1
  Integrator3/1 -> Out1/1, Sum12/2
  In1/1 -> Sum12/1
  Gain2/1 -> Sum13/1
  Gain5/1 -> Integrator2/1
  Sum13/1 -> Gain5/1
  Gain8/1 -> Sum13/2
  Integrator2/1 -> Gain7/1, Integrator3/1

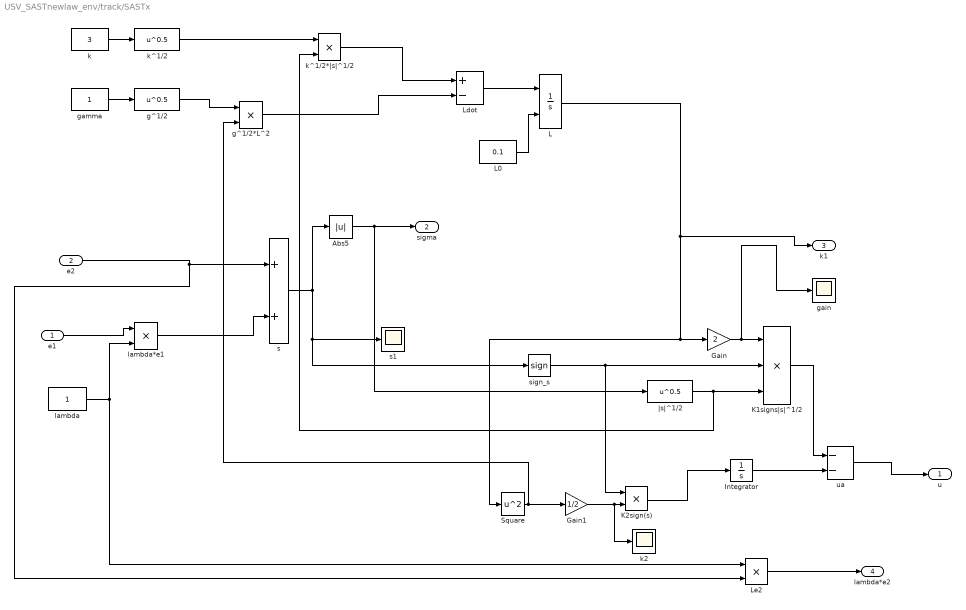
== system USV_SASTnewlaw_env/track/SASTx ==
  e1 : Inport
  e2 : Inport  Port=2
  Abs5 : Abs  SaturateOnIntegerOverflow=off
  Gain : Gain  Gain=2
  Gain1 : Gain  Gain=1/2
  Integrator : Integrator
  K1signs|s|^1/2 : Product  Inputs=***
  K2sign(s) : Product
  L : Integrator  InitialConditionSource=external
  L0 : Constant  Value=0.1
  Ldot : Sum  Inputs=+-
  Le2 : Product
  Square : Math  Operator=square
  g^1/2 : Fcn  Expr=u^0.5
  g^1/2*L^2 : Product
  gain : Scope
  gamma : Constant
  k : Constant  Value=3
  k2 : Scope
  k^1/2 : Fcn  Expr=u^0.5
  k^1/2*|s|^1/2 : Product
  lambda : Constant
  lambda*e1 : Product
  s : Sum
  s1 : Scope
  sign_s : Signum
  ua : Sum  Inputs=--
  |s|^1/2 : Fcn  Expr=u^0.5
  u : Outport  VectorParamsAs1DForOutWhenUnconnected=off
  sigma : Outport  Port=2  VectorParamsAs1DForOutWhenUnconnected=off
  k1 : Outport  Port=3  VectorParamsAs1DForOutWhenUnconnected=off
  lambda*e2 : Outport  Port=4  VectorParamsAs1DForOutWhenUnconnected=off
  wires:
  s/1 -> s1/1, sign_s/1, Abs5/1
  sign_s/1 -> K2sign(s)/1, K1signs|s|^1/2/2
  K1signs|s|^1/2/1 -> ua/1
  Abs5/1 -> |s|^1/2/1, sigma/1
  |s|^1/2/1 -> k^1/2*|s|^1/2/2, K1signs|s|^1/2/3
  Le2/1 -> lambda*e2/1
  e2/1 -> Le2/2, s/1
  lambda/1 -> Le2/1, lambda*e1/2
  e1/1 -> lambda*e1/1
  lambda*e1/1 -> s/2
  L/1 -> k1/1, Gain/1, Square/1
  ua/1 -> u/1
  Gain/1 -> gain/1, K1signs|s|^1/2/1
  Integrator/1 -> ua/2
  K2sign(s)/1 -> Integrator/1
  Square/1 -> g^1/2*L^2/2, Gain1/1
  Gain1/1 -> k2/1, K2sign(s)/2
  Ldot/1 -> L/1
  L0/1 -> L/2
  k/1 -> k^1/2/1
  gamma/1 -> g^1/2/1
  g^1/2/1 -> g^1/2*L^2/1
  k^1/2/1 -> k^1/2*|s|^1/2/1
  g^1/2*L^2/1 -> Ldot/2
  k^1/2*|s|^1/2/1 -> Ldot/1

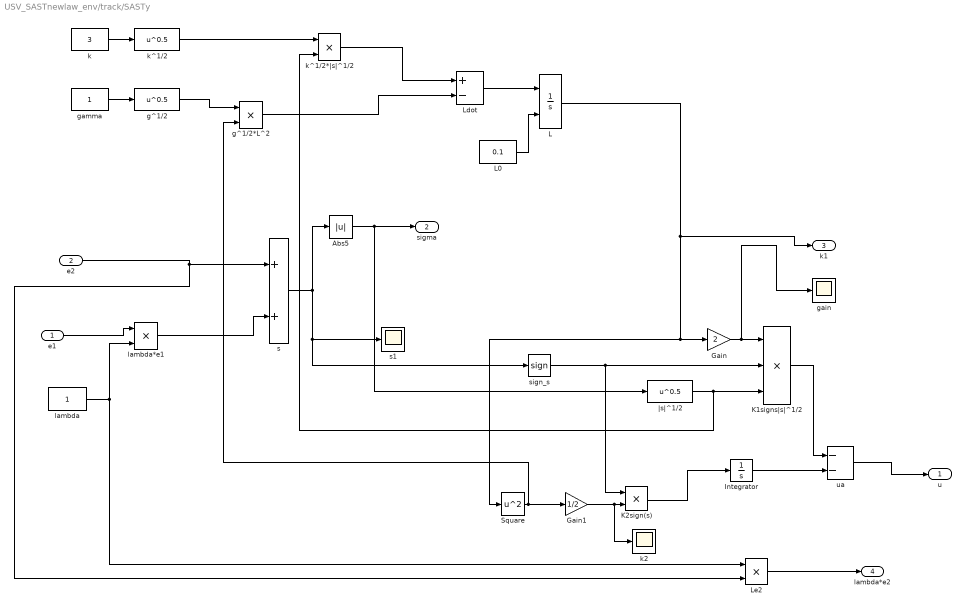
== system USV_SASTnewlaw_env/track/SASTy ==
  e1 : Inport
  e2 : Inport  Port=2
  Abs5 : Abs  SaturateOnIntegerOverflow=off
  Gain : Gain  Gain=2
  Gain1 : Gain  Gain=1/2
  Integrator : Integrator
  K1signs|s|^1/2 : Product  Inputs=***
  K2sign(s) : Product
  L : Integrator  InitialConditionSource=external
  L0 : Constant  Value=0.1
  Ldot : Sum  Inputs=+-
  Le2 : Product
  Square : Math  Operator=square
  g^1/2 : Fcn  Expr=u^0.5
  g^1/2*L^2 : Product
  gain : Scope
  gamma : Constant
  k : Constant  Value=3
  k2 : Scope
  k^1/2 : Fcn  Expr=u^0.5
  k^1/2*|s|^1/2 : Product
  lambda : Constant
  lambda*e1 : Product
  s : Sum
  s1 : Scope
  sign_s : Signum
  ua : Sum  Inputs=--
  |s|^1/2 : Fcn  Expr=u^0.5
  u : Outport  VectorParamsAs1DForOutWhenUnconnected=off
  sigma : Outport  Port=2  VectorParamsAs1DForOutWhenUnconnected=off
  k1 : Outport  Port=3  VectorParamsAs1DForOutWhenUnconnected=off
  lambda*e2 : Outport  Port=4  VectorParamsAs1DForOutWhenUnconnected=off
  wires:
  s/1 -> s1/1, sign_s/1, Abs5/1
  sign_s/1 -> K2sign(s)/1, K1signs|s|^1/2/2
  K1signs|s|^1/2/1 -> ua/1
  Abs5/1 -> |s|^1/2/1, sigma/1
  |s|^1/2/1 -> k^1/2*|s|^1/2/2, K1signs|s|^1/2/3
  Le2/1 -> lambda*e2/1
  e2/1 -> Le2/2, s/1
  lambda/1 -> Le2/1, lambda*e1/2
  e1/1 -> lambda*e1/1
  lambda*e1/1 -> s/2
  L/1 -> k1/1, Gain/1, Square/1
  ua/1 -> u/1
  Gain/1 -> gain/1, K1signs|s|^1/2/1
  Integrator/1 -> ua/2
  K2sign(s)/1 -> Integrator/1
  Square/1 -> g^1/2*L^2/2, Gain1/1
  Gain1/1 -> k2/1, K2sign(s)/2
  Ldot/1 -> L/1
  L0/1 -> L/2
  k/1 -> k^1/2/1
  gamma/1 -> g^1/2/1
  g^1/2/1 -> g^1/2*L^2/1
  k^1/2/1 -> k^1/2*|s|^1/2/1
  g^1/2*L^2/1 -> Ldot/2
  k^1/2*|s|^1/2/1 -> Ldot/1

== system USV_SASTnewlaw_env/USV_Env/Currents/w ==
  Demux : Demux  Tag=STV Demux  Outputs=3
      settings: DisplayOption=none
  FromWs : FromWorkspace  Tag=STV FromWs  VariableName=tuvar
      SigBuilderData=|
      | common.afterFinalStr = 'Extrapolate'
      | common.sampleTime = 0
      | dataSet.timeRange = [0 200]
      | dataSet.name = 'Group 1'
      | sbobj.Groups.Name = 'Group 1'
      | sbobj.Groups.Signals(1).Name = 'white_noise'
      | sbobj.Groups.Signals(1).XData = [0 0.05 0.1 0.15 0.2 0.25 0.3 0.35 0.4 0.45 0.5 0.55 ... (4001 elements, 1x4001)]
      | sbobj.Groups.Signals(1).YData = [1.30023943573 1.08515455929 -0.452245973079 1.83154112912 1.15232545779 0.288810864745 -0.42626545614 0.320042144717 1.64242738525 -0.789338506726 -0.925024019679 0.348861046149 ... (4001 elements, 1x4001)]
      | sbobj.Groups.Signals(2).Name = '0.4'
      | sbobj.Groups.Signals(2).XData = [0 200]
      | sbobj.Groups.Signals(2).YData = [0.4 0.4]
      | sbobj.Groups.Signals(3).Name = 'zero'
      | sbobj.Groups.Signals(3).XData = [0 200]
      | sbobj.Groups.Signals(3).YData = [0 0]
      | sbobj.Groups.TimeRange = [0 200]
  white_noise : Outport  Tag=STV Outport
  0.4 : Outport  Tag=STV Outport  Port=2
  zero : Outport  Tag=STV Outport  Port=3
  wires:
  Demux/1 -> white_noise/1
  FromWs/1 -> Demux/1
  Demux/2 -> 0.4/1
  Demux/3 -> zero/1

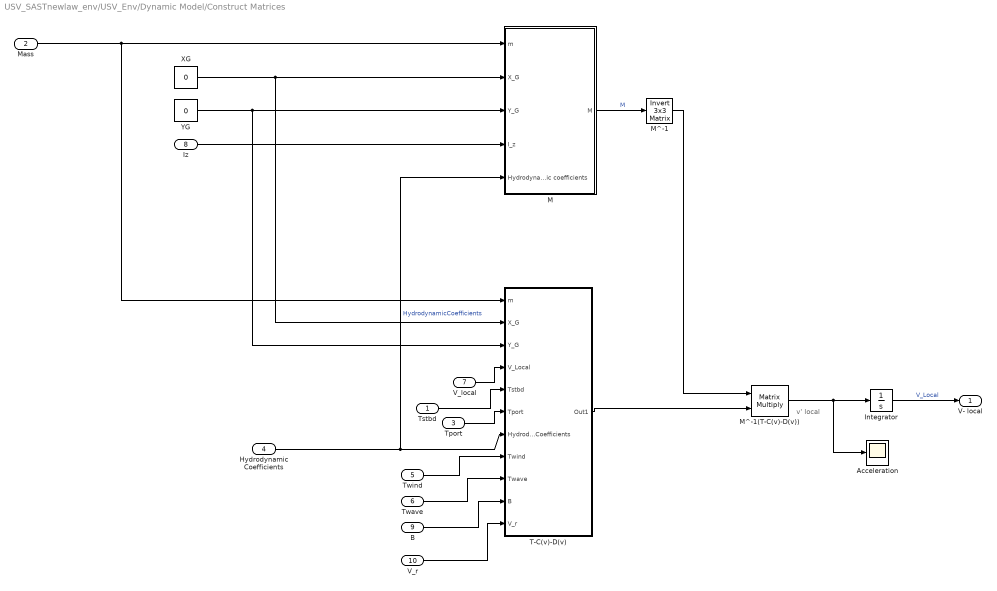
== system USV_SASTnewlaw_env/USV_Env/Dynamic Model/Construct Matrices ==
  note: v' local
  Tstbd : Inport
  "Mass " : Inport  Port=2
  Tport : Inport  Port=3
  Hydrodynamic Coefficients : Inport  Port=4
  Twind : Inport  Port=5
  Twave : Inport  Port=6
  V_local : Inport  Port=7
  Iz : Inport  Port=8
  B : Inport  Port=9
  V_r : Inport  Port=10
  Acceleration : Scope
  Integrator : Integrator
  M : Subsystem
  M^-1 : aerolibutil/Invert  3x3 Matrix
  M^-1(T-C(v)-D(v)) : Product  Multiplication=Matrix(*)
  T-C(v)-D(v) : Subsystem
  XG : Constant  Value=0
  YG : Constant  Value=0
  V- local : Outport  VectorParamsAs1DForOutWhenUnconnected=off
  wires:
  M/1(M) -> M^-1/1  "M"
  Integrator/1 -> V- local/1  "V_Local"
  M^-1(T-C(v)-D(v))/1 -> Acceleration/1, Integrator/1
  Iz/1 -> M/4(I_z)
  M^-1/1 -> M^-1(T-C(v)-D(v))/1
  Hydrodynamic Coefficients/1 -> M/5(Hydrodynamic coefficients), T-C(v)-D(v)/7(HydrodynamicCoefficients)  "HydrodynamicCoefficients"
  YG/1 -> T-C(v)-D(v)/3(Y_G), M/3(Y_G)
  "Mass "/1 -> T-C(v)-D(v)/1(m), M/1(m)
  XG/1 -> T-C(v)-D(v)/2(X_G), M/2(X_G)
  Tstbd/1 -> T-C(v)-D(v)/5(Tstbd)
  Tport/1 -> T-C(v)-D(v)/6(Tport)
  T-C(v)-D(v)/1(Out1) -> M^-1(T-C(v)-D(v))/2
  Twave/1 -> T-C(v)-D(v)/9(Twave)
  Twind/1 -> T-C(v)-D(v)/8(Twind)
  V_local/1 -> T-C(v)-D(v)/4(V_Local)
  B/1 -> T-C(v)-D(v)/10(B)
  V_r/1 -> T-C(v)-D(v)/11(V_r)

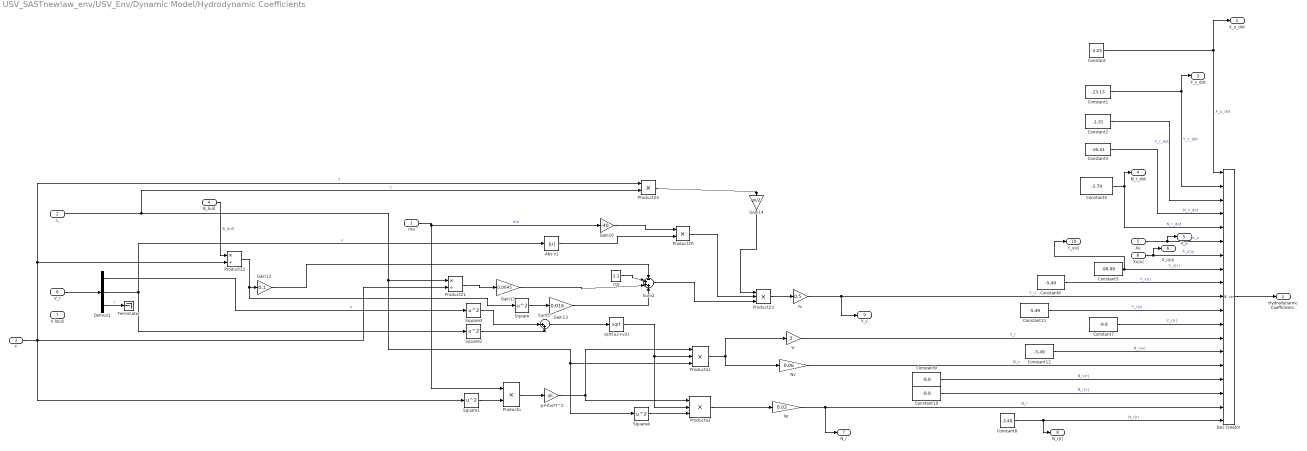
== system USV_SASTnewlaw_env/USV_Env/Dynamic Model/Hydrodynamic Coefficients ==
  rho : Inport
  L : Inport  Port=2
  T : Inport  Port=3
  B_hull : Inport  Port=4
  Xu : Inport  Port=5
  Xu|u| : Inport  Port=6
  V local : Inport  Port=7
  V_r : Inport  Port=8
  -pi*rho*T^2 : Gain  Gain=-pi
  Abs v1 : Abs  SaturateOnIntegerOverflow=off
  Bus Creator : BusCreator  Inputs=19
  Constant : Constant  Value=-2.25
  Constant1 : Constant  Value=-23.13
  Constant10 : Constant  Value=-8.8
  Constant11 : Constant  Value=-5.49
  Constant12 : Constant  Value=-5.49
  Constant2 : Constant  Value=-1.31
  Constant3 : Constant  Value=-16.41
  Constant4 : Constant  Value=-2.79
  Constant5 : Constant  Value=-99.99
  Constant6 : Constant  Value=-5.49
  Constant7 : Constant  Value=-8.8
  Constant8 : Constant  Value=-3.49
  Constant9 : Constant  Value=-8.8
  Demux1 : Demux  Outputs=3
  Gain10 : Gain  Gain=-40
  Gain11 : Gain  Gain=0.0045
  Gain12 : Gain  Gain=0.1
  Gain13 : Gain  Gain=0.016
  Gain14 : Gain  Gain=pi/2
  Nr : Gain  Gain=0.02
  Nv : Gain  Gain=0.06
  Product20 : Product
  Product21 : Product  Inputs=*/
  Product22 : Product  Inputs=*/
  Product23 : Product  Inputs=3
  Product24 : Product
  Producto : Product
  Producto1 : Product  Inputs=3
  Producto2 : Product  Inputs=3
  Square{,1..4} (5 alike) : Math  Operator=square  SignedPower=on
  Sum2 : Sum  Inputs=-+++
  Sum5 : Sum  Inputs=|++
  Terminator : Terminator
  Yr : Gain  Gain=3
  Yv : Gain  Gain=0.5
  cte : Constant  Value=1.1
  sqrt(u2+v2) : Sqrt
  "Hydrodynamic Coefficients " : Outport  VectorParamsAs1DForOutWhenUnconnected=off
  X_u_dot : Outport  Port=2  VectorParamsAs1DForOutWhenUnconnected=off
  Y_v_dot : Outport  Port=3  VectorParamsAs1DForOutWhenUnconnected=off
  N_r_dot : Outport  Port=4  VectorParamsAs1DForOutWhenUnconnected=off
  X_u : Outport  Port=5  VectorParamsAs1DForOutWhenUnconnected=off
  X_u|u| : Outport  Port=6  VectorParamsAs1DForOutWhenUnconnected=off
  N_r : Outport  Port=7  VectorParamsAs1DForOutWhenUnconnected=off
  N_r|r| : Outport  Port=8  VectorParamsAs1DForOutWhenUnconnected=off
  Y_v : Outport  Port=9  VectorParamsAs1DForOutWhenUnconnected=off
  Y_v|v| : Outport  Port=10  VectorParamsAs1DForOutWhenUnconnected=off
  wires:
  Constant3/1 -> Bus Creator/4  "N_v_dot"
  Constant/1 -> X_u_dot/1, Bus Creator/1  "X_u_dot"
  Square/1 -> Gain13/1
  Gain14/1 -> Product23/1
  Product24/1 -> Gain14/1
  Square4/1 -> Producto2/3
  sqrt(u2+v2)/1 -> Producto2/2, Producto1/2
  Product20/1 -> Product23/2
  Gain13/1 -> Sum2/4
  B_hull/1 -> Product22/1  "B_hull"
  Square2/1 -> Sum5/2
  Gain12/1 -> Sum2/1
  Sum2/1 -> Product23/3
  Gain10/1 -> Product20/1
  Product23/1 -> Yv/1
  cte/1 -> Sum2/2
  Constant2/1 -> Bus Creator/3  "Y_r_dot"
  Gain11/1 -> Sum2/3
  Square1/1 -> Producto/2
  Producto2/1 -> Nr/1
  Square3/1 -> Sum5/1
  Sum5/1 -> sqrt(u2+v2)/1
  rho/1 -> Producto/1, Gain10/1  "rho"
  Abs v1/1 -> Product20/2
  Product21/1 -> Gain11/1
  Producto1/1 -> Yr/1, Nv/1
  Product22/1 -> Square/1, Gain12/1
  Producto/1 -> -pi*rho*T^2/1
  -pi*rho*T^2/1 -> Producto1/1, Producto2/1
  T/1 -> Product24/1, Product22/2, Square1/1, Product21/2  "T"
  L/1 -> Square4/1, Producto1/3, Product21/1, Product24/2  "L"
  Nv/1 -> Bus Creator/15  "N_v"
  Constant5/1 -> Y_v|v|/1, Bus Creator/8  "Y_v|v|"
  Yv/1 -> Y_v/1, Bus Creator/10  "Y_v"
  Constant6/1 -> Bus Creator/9  "Y_v|r|"
  Yr/1 -> Bus Creator/13  "Y_r"
  Constant8/1 -> N_r|r|/1, Bus Creator/19  "N_r|r|"
  Nr/1 -> Bus Creator/18, N_r/1  "N_r"
  Xu|u|/1 -> X_u|u|/1, Bus Creator/7  "X_u|u|"
  Constant7/1 -> Bus Creator/12  "Y_r|r|"
  Xu/1 -> X_u/1, Bus Creator/6  "X_u"
  Bus Creator/1 -> "Hydrodynamic Coefficients "/1
  Constant4/1 -> Bus Creator/5, N_r_dot/1  "N_r_dot"
  Constant1/1 -> Y_v_dot/1, Bus Creator/2  "Y_v_dot"
  Demux1/1 -> Square3/1  "u"
  V_r/1 -> Demux1/1
  Demux1/2 -> Square2/1, Abs v1/1  "v"
  Demux1/3 -> Terminator/1  "r"
  Constant10/1 -> Bus Creator/17  "N_r|v|"
  Constant9/1 -> Bus Creator/16  "N_v|r|"
  Constant12/1 -> Bus Creator/14  "N_v|v|"
  Constant11/1 -> Bus Creator/11  "Y_r|v|"

== system USV_SASTnewlaw_env/USV_Env/Dynamic Model/Subsystem5 ==
  psi : Inport
  " J(n)" : sharedutil/Create 3x3 Matrix  aMode=aMode
  Constant1 : Constant
  Constant2 : Constant  Value=0
  Gain9 : Gain  Gain=-1
  Selector : Selector  InputPortWidth=3  IndexOptions=Index vector (dialog)  Indices=3  OutputSizes=1
  Trigonometric Function : Trigonometry
  Trigonometric Function1 : Trigonometry  Operator=cos
  J(n) : Outport  VectorParamsAs1DForOutWhenUnconnected=off
  wires:
  Gain9/1 -> " J(n)"/2
  Trigonometric Function1/1 -> " J(n)"/5, " J(n)"/1
  Trigonometric Function/1 -> " J(n)"/4, Gain9/1
  Constant1/1 -> " J(n)"/9
  psi/1 -> Selector/1
  " J(n)"/1 -> J(n)/1
  Constant2/1 -> " J(n)"/8, " J(n)"/7, " J(n)"/6, " J(n)"/3
  Selector/1 -> Trigonometric Function1/1, Trigonometric Function/1

== system USV_SASTnewlaw_env/USV_Env/Dynamic Model/VCrurrent - local ==
  psi : Inport
  BetaCurrent : Inport  Port=2
  VC : Inport  Port=3
  Demux1 : Demux  Outputs=3
  Mux1 : Mux  Inputs=3
  Product1 : Product
  Product2 : Product
  Sum7 : Sum  Inputs=|+-
  Terminator : Terminator
  Terminator1 : Terminator
  Trigonometric Function : Trigonometry
  Trigonometric Function1 : Trigonometry  Operator=cos
  rc : Constant  Value=0
  VCurrent - local : Outport  VectorParamsAs1DForOutWhenUnconnected=off
  wires:
  psi/1 -> Demux1/1
  Sum7/1 -> Trigonometric Function/1, Trigonometric Function1/1
  BetaCurrent/1 -> Sum7/1
  Demux1/3 -> Sum7/2
  Trigonometric Function/1 -> Product1/2
  Trigonometric Function1/1 -> Product2/1
  Demux1/2 -> Terminator1/1  "y"
  Demux1/1 -> Terminator/1  "x"
  Mux1/1 -> VCurrent - local/1
  Product2/1 -> Mux1/1
  Product1/1 -> Mux1/2
  VC/1 -> Product1/1, Product2/2
  rc/1 -> Mux1/3

== system USV_SASTnewlaw_env/USV_Env/Waves/Fwave ==
  we : Inport
  lambda : Inport  Port=2
  Kw : Gain  Gain=0.64
  Product : Product
  Product1 : Product  Inputs=3
  Saturation : Saturate  UpperLimit=20  LowerLimit=-20
  Square : Math  Operator=square
  Sum : Sum
  Sum1 : Sum  Inputs=--+
  Wave Force : Scope  NumInputPorts=2
  Xw1 yw : Integrator
  Xw2 : Integrator
  d : Integrator
  gain : Gain  Gain=2
  w : Subsystem  Tag=STV Subsys  LoadFcn=sigbuilder_block('load');  StartFcn=sigbuilder_block('start');  StopFcn=sigbuilder_block('stop');  ClipboardFcn=sigbuilder_block('clipboard');  mask(Sigbuilder block){tuvar=[0:10]}
      mask help: Simulink:masks:SigbuilderBlock_MD
      mask init:
      | if ~strcmp(get_param(bdroot(gcbh),'SimulationStatus'),'stopped') tuvar = sigbuilder_block('maskInit'); end
      settings: CopyFcn=sigbuilder_block('copy');  DeleteFcn=sigbuilder_block('delete');  ModelCloseFcn=sigbuilder_block('modelClose');  PreSaveFcn=sigbuilder_block('preSave');  PauseFcn=sigbuilder_block('pause');  ContinueFcn=sigbuilder_block('continue');  NameChangeFcn=sigbuilder_block('namechange');  OpenFcn=sigbuilder_block('open',[1614 67.5 717 628.5 ]);  CloseFcn=sigbuilder_block('close');
      mask Display: plot(0, 0, 100, 100,[2, 2, 32, 32, 2], [68, 8, 8, 68, 68],[32, 2], [38, 38], [32, 19, 2],[53, 60, 44], [32, 17, 17, 2],[16, 16, 31, 31]);txt = getActiveGroup(gcbh);text(2, 100, txt,'verticalAlignment', 'top');
  Xwave : Outport  VectorParamsAs1DForOutWhenUnconnected=off
  wires:
  w/2(d) -> d/1
  Xw1 yw/1 -> Product/2, Wave Force/1, Sum/1
  Product/1 -> Sum1/2
  Kw/1 -> Sum1/3
  gain/1 -> Sum1/1
  Sum/1 -> Xwave/1
  Product1/1 -> gain/1
  d/1 -> Saturation/1
  Sum1/1 -> Xw2/1
  we/1 -> Product1/3, Square/1
  lambda/1 -> Product1/2
  Square/1 -> Product/1
  Xw2/1 -> Product1/1, Xw1 yw/1
  Saturation/1 -> Wave Force/2, Sum/2
  w/1(w) -> Kw/1

== system USV_SASTnewlaw_env/USV_Env/Waves/N ==
  we : Inport
  lambda : Inport  Port=2
  Kw : Gain  Gain=0.64
  Product : Product
  Product1 : Product  Inputs=3
  Saturation : Saturate  UpperLimit=5  LowerLimit=-5
  Square : Math  Operator=square
  Sum : Sum
  Sum1 : Sum  Inputs=--+
  Xw1 yw : Integrator
  Xw2 : Integrator
  d : Integrator
  gain : Gain  Gain=2
  w : Subsystem  Tag=STV Subsys  LoadFcn=sigbuilder_block('load');  StartFcn=sigbuilder_block('start');  StopFcn=sigbuilder_block('stop');  ClipboardFcn=sigbuilder_block('clipboard');  mask(Sigbuilder block){tuvar=[0:10]}
      mask help: Simulink:masks:SigbuilderBlock_MD
      mask init:
      | if ~strcmp(get_param(bdroot(gcbh),'SimulationStatus'),'stopped') tuvar = sigbuilder_block('maskInit'); end
      settings: CopyFcn=sigbuilder_block('copy');  DeleteFcn=sigbuilder_block('delete');  ModelCloseFcn=sigbuilder_block('modelClose');  PreSaveFcn=sigbuilder_block('preSave');  PauseFcn=sigbuilder_block('pause');  ContinueFcn=sigbuilder_block('continue');  NameChangeFcn=sigbuilder_block('namechange');  OpenFcn=sigbuilder_block('open',[109.5 26.25 710.25 647.25 ]);  CloseFcn=sigbuilder_block('close');
      mask Display: plot(0, 0, 100, 100,[2, 2, 32, 32, 2], [68, 8, 8, 68, 68],[32, 2], [38, 38], [32, 19, 2],[53, 60, 44], [32, 17, 17, 2],[16, 16, 31, 31]);txt = getActiveGroup(gcbh);text(2, 100, txt,'verticalAlignment', 'top');
  Nwave : Outport  VectorParamsAs1DForOutWhenUnconnected=off
  wires:
  Xw1 yw/1 -> Product/2, Sum/1
  Product/1 -> Sum1/2
  Kw/1 -> Sum1/3
  gain/1 -> Sum1/1
  Sum/1 -> Nwave/1
  Product1/1 -> gain/1
  d/1 -> Saturation/1
  Sum1/1 -> Xw2/1
  we/1 -> Product1/3, Square/1
  lambda/1 -> Product1/2
  Square/1 -> Product/1
  Xw2/1 -> Product1/1, Xw1 yw/1
  Saturation/1 -> Sum/2
  w/2(d) -> d/1
  w/1(w) -> Kw/1

== system USV_SASTnewlaw_env/USV_Env/Waves/we ==
  psi : Inport
  u : Inport  Port=2
  v : Inport  Port=3
  wave_beta : Inport  Port=4
  1/g : Gain  Gain=1/9.81
  Abs : Abs  SaturateOnIntegerOverflow=off
  Product1 : Product  Inputs=3
  Square : Math  Operator=square
  Square1 : Math  Operator=square
  Square2 : Math  Operator=square
  Sum1 : Sum  Inputs=+-
  Sum2 : Sum
  Sum3 : Sum  Inputs=+-
  Trigonometric Function1 : Trigonometry  Operator=cos
  U : Sqrt
  w0 : Constant  Value=0.8
  w : Outport  VectorParamsAs1DForOutWhenUnconnected=off
  wires:
  u/1 -> Square/1
  v/1 -> Square1/1
  Square1/1 -> Sum2/1
  Square/1 -> Sum2/2
  Sum2/1 -> U/1
  Square2/1 -> 1/g/1
  w0/1 -> Sum3/1, Square2/1
  1/g/1 -> Product1/1
  U/1 -> Product1/2
  Product1/1 -> Sum3/2
  Sum3/1 -> Abs/1
  Abs/1 -> w/1
  psi/1 -> Sum1/1
  wave_beta/1 -> Sum1/2
  Sum1/1 -> Trigonometric Function1/1
  Trigonometric Function1/1 -> Product1/3

== system USV_SASTnewlaw_env/USV_Env/Wind/C_N ==
  CY : Inport
  gammarw : Inport  Port=2
  -0.18 : Gain  Gain=-0.18
  Product : Product
  Sum3 : Sum  Inputs=|+-
  pi/2 : Constant  Value=pi/2
  CN : Outport  VectorParamsAs1DForOutWhenUnconnected=off
  wires:
  gammarw/1 -> Sum3/1
  -0.18/1 -> Product/2
  Product/1 -> CN/1
  CY/1 -> Product/1
  Sum3/1 -> -0.18/1
  pi/2/1 -> Sum3/2

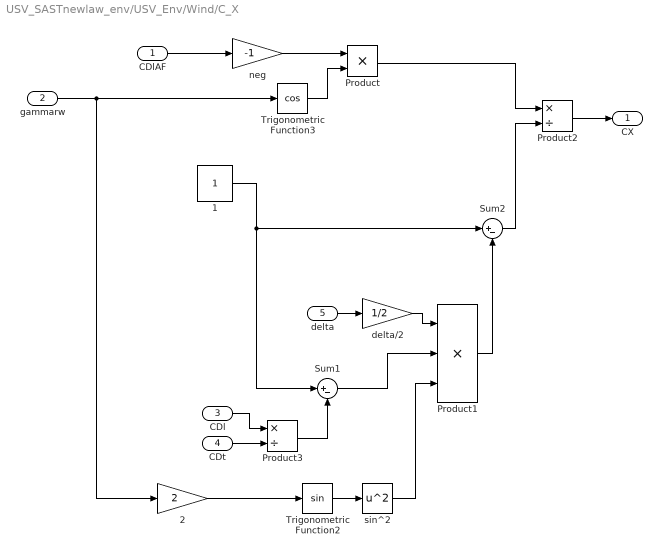
== system USV_SASTnewlaw_env/USV_Env/Wind/C_X ==
  CDlAF : Inport
  gammarw : Inport  Port=2
  CDl : Inport  Port=3
  CDt : Inport  Port=4
  delta : Inport  Port=5
  1 : Constant
  2 : Gain  Gain=2
  Product : Product
  Product1 : Product  Inputs=***
  Product2 : Product  Inputs=*/
  Product3 : Product  Inputs=*/
  Sum1 : Sum  Inputs=|+-
  Sum2 : Sum  Inputs=|+-
  Trigonometric Function2 : Trigonometry
  Trigonometric Function3 : Trigonometry  Operator=cos
  delta/2 : Gain  Gain=1/2
  neg : Gain  Gain=-1
  sin^2 : Math  Operator=square
  CX : Outport  VectorParamsAs1DForOutWhenUnconnected=off
  wires:
  gammarw/1 -> 2/1, Trigonometric Function3/1
  CDlAF/1 -> neg/1
  Trigonometric Function3/1 -> Product/2
  1/1 -> Sum1/1, Sum2/1
  Product1/1 -> Sum2/2
  delta/1 -> delta/2/1
  delta/2/1 -> Product1/1
  Product/1 -> Product2/1
  Sum2/1 -> Product2/2
  Product2/1 -> CX/1
  Product3/1 -> Sum1/2
  CDt/1 -> Product3/2
  CDl/1 -> Product3/1
  Trigonometric Function2/1 -> sin^2/1
  2/1 -> Trigonometric Function2/1
  sin^2/1 -> Product1/3
  Sum1/1 -> Product1/2
  neg/1 -> Product/1

== system USV_SASTnewlaw_env/USV_Env/Wind/C_Y ==
  gammarw : Inport
  CDl : Inport  Port=2
  CDt : Inport  Port=3
  delta : Inport  Port=4
  1 : Constant
  2 : Gain  Gain=2
  Product : Product
  Product1 : Product  Inputs=***
  Product2 : Product  Inputs=*/
  Product3 : Product  Inputs=*/
  Sum1 : Sum  Inputs=|+-
  Sum2 : Sum  Inputs=|+-
  Trigonometric Function2 : Trigonometry
  Trigonometric Function3 : Trigonometry
  delta/2 : Gain  Gain=1/2
  sin^2 : Math  Operator=square
  CY : Outport  VectorParamsAs1DForOutWhenUnconnected=off
  wires:
  gammarw/1 -> 2/1, Trigonometric Function3/1
  Trigonometric Function3/1 -> Product/1
  1/1 -> Sum1/1, Sum2/1
  Product1/1 -> Sum2/2
  delta/1 -> delta/2/1
  delta/2/1 -> Product1/1
  Product/1 -> Product2/1
  Sum2/1 -> Product2/2
  Product2/1 -> CY/1
  Product3/1 -> Sum1/2
  CDt/1 -> Product3/2, Product/2
  CDl/1 -> Product3/1
  Trigonometric Function2/1 -> sin^2/1
  2/1 -> Trigonometric Function2/1
  sin^2/1 -> Product1/3
  Sum1/1 -> Product1/2

== system USV_SASTnewlaw_env/USV_Env/Wind/Vw ==
  Demux : Demux  Tag=STV Demux
      settings: DisplayOption=none
  FromWs : FromWorkspace  Tag=STV FromWs  VariableName=tuvar
      SigBuilderData=|
      | common.afterFinalStr = 'Extrapolate'
      | common.sampleTime = 0
      | dataSet.timeRange = [0 200]
      | dataSet.name = 'Group 1'
      | sbobj.Groups.Name = 'Group 1'
      | sbobj.Groups.Signals(1).Name = 'Gentle Breeze'
      | sbobj.Groups.Signals(1).XData = [0 200]
      | sbobj.Groups.Signals(1).YData = [5.11 5.11]
      | sbobj.Groups.Signals(2).Name = 'Moderate Breeze'
      | sbobj.Groups.Signals(2).XData = [0 200]
      | sbobj.Groups.Signals(2).YData = [7.2 7.2]
      | sbobj.Groups.Signals(3).Name = 'Fresh Breeze'
      | sbobj.Groups.Signals(3).XData = [0 200]
      | sbobj.Groups.Signals(3).YData = [10.28 10.28]
      | sbobj.Groups.Signals(4).Name = 'Calm (0)'
      | sbobj.Groups.Signals(4).XData = [0 200]
      | sbobj.Groups.Signals(4).YData = [0 0]
      | sbobj.Groups.TimeRange = [0 200]
  Gentle Breeze : Outport  Tag=STV Outport
  Moderate Breeze : Outport  Tag=STV Outport  Port=2
  Fresh Breeze : Outport  Tag=STV Outport  Port=3
  Calm (0) : Outport  Tag=STV Outport  Port=4
  wires:
  Demux/1 -> Gentle Breeze/1
  FromWs/1 -> Demux/1
  Demux/2 -> Moderate Breeze/1
  Demux/3 -> Fresh Breeze/1
  Demux/4 -> Calm (0)/1
